simulink model "ex3"  (R2020a)
settings: Solver=ode45  StartTime=0.0  StopTime=8  RelTol=1e-3  EnableMultiTasking=on
values from neighbouring files (symbols this model uses):
  A = gss.a    [ex3.m]
  B = gss.b    [ex3.m]
  C = gss.c    [ex3.m]
  K = place(Aa,Ba,[-4 -5 -7])    [ex3.m]
  L = place(A',C',obsepoles)'    [ex3.m]
settings Model: Creator=Xrisostomos  LastModifiedBy=xriso
settings DataIOCC: LimitDataPoints=on  SaveFormat=Array  ReturnWorkspaceOutputs=off
settings OptimizationCC: LifeSpan=inf
settings DebuggingCC: SFUnexpectedBacktrackingDiag=warning  SFNoUnconditionalDefaultTransitionDiag=warning  SFExecutionAtInitializationDiag=none  ArithmeticOperatorsInVariantConditions=warning
settings HardwareCC: ProdBitPerPointer=32  ProdBitPerSizeT=32  ProdBitPerPtrDiffT=32  ProdLargestAtomicFloat=None  ProdIntDivRoundTo=Undefined  ProdEndianess=Unspecified  ProdWordSize=32  ProdHWDeviceType=32-bit Generic
settings ModelReferenceCC: PropagateSignalLabelsOutOfModel=off
settings SFSimCC: SimUseLocalCustomCode=off  CustomCodeUndefinedFunction=UseInterfaceOnly
settings RTWCC: RTWUseLocalCustomCode=off
settings CodeAppCC: StateflowObjectComments=on
settings GRTTargetCC: TargetLangStandard=C89/C90 (ANSI)
settings ConfigComp: CovMetricSettings=dw  CovHtmlReporting=on  CovSaveCumulativeToWorkspaceVar=on  CovSaveSingleToWorkspaceVar=on  CovExternalEMLEnable=off

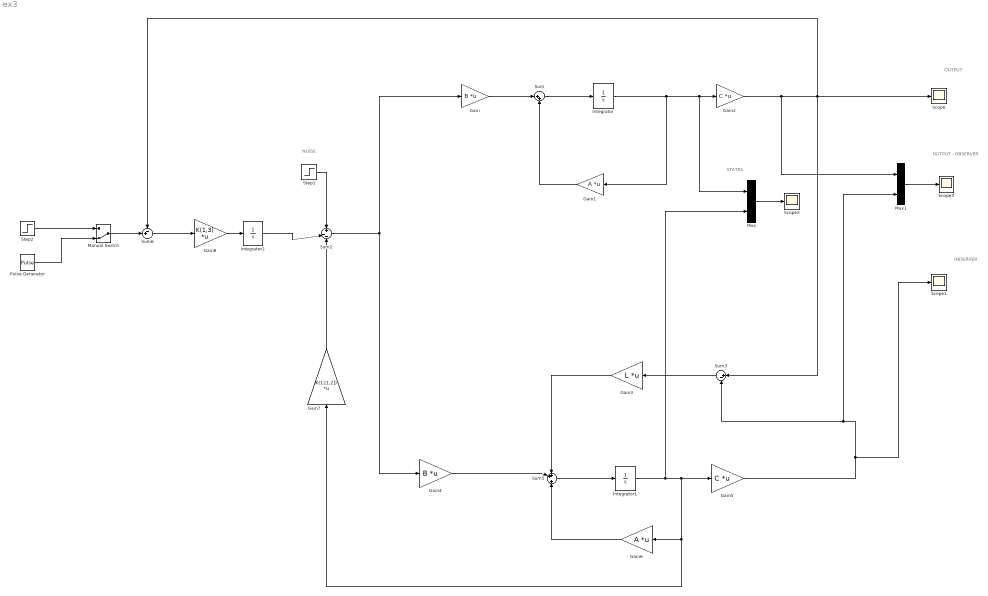
== system ex3 ==
  note: NOISE
  note: OUTPUT
  note: OBSERVER
  note: OUTPUT - OBSERVER
  note: STATES
  Gain : Gain  Gain=B  Multiplication=Matrix(K*u)
  Gain1 : Gain  Gain=A  Multiplication=Matrix(K*u)
  Gain2 : Gain  Gain=C  Multiplication=Matrix(K*u)
  Gain3 : Gain  Gain=L  Multiplication=Matrix(K*u)
  Gain4 : Gain  Gain=B  Multiplication=Matrix(K*u)
  Gain5 : Gain  Gain=C  Multiplication=Matrix(K*u)
  Gain6 : Gain  Gain=A  Multiplication=Matrix(K*u)
  Gain7 : Gain  Gain=K(1,[1,2])  Multiplication=Matrix(K*u)
  Gain8 : Gain  Gain=K(1,3)  Multiplication=Matrix(K*u)
  Integrator : Integrator  InitialCondition=[1 1]
  Integrator1 : Integrator  InitialCondition=[0 0]
  Integrator2 : Integrator
  Manual Switch : ManualSwitch  CurrentSetting=0
  Mux : Mux  Inputs=2
  Mux1 : Mux  Inputs=2
  Pulse Generator : DiscretePulseGenerator  PulseType=Time based  Period=4  PulseWidth=50
  Scope{,1..3} (4 alike) : Scope
  Step1 : Step  Time=5  SampleTime=0
  Step2 : Step  SampleTime=0
  Sum : Sum  Inputs=|++
  Sum2 : Sum  Inputs=+|--
  Sum3 : Sum  Inputs=|+-
  Sum5 : Sum  Inputs=++|+
  Sum6 : Sum  Inputs=-+|
  wires:
  Gain/1 -> Sum/1
  Sum/1 -> Integrator/1
  Integrator/1 -> Mux/1, Gain2/1, Gain1/1
  Gain1/1 -> Sum/2
  Gain3/1 -> Sum5/1
  Sum3/1 -> Gain3/1
  Gain5/1 -> Mux1/2, Sum3/2, Scope1/1
  Gain4/1 -> Sum5/2
  Sum5/1 -> Integrator1/1
  Gain6/1 -> Sum5/3
  Integrator1/1 -> Mux/2, Gain6/1, Gain7/1, Gain5/1
  Sum2/1 -> Gain/1, Gain4/1
  Gain7/1 -> Sum2/3
  Integrator2/1 -> Sum2/2
  Gain8/1 -> Integrator2/1
  Gain2/1 -> Mux1/1, Scope/1, Sum3/1, Sum6/1
  Sum6/1 -> Gain8/1
  Mux/1 -> Scope2/1
  Step1/1 -> Sum2/1
  Mux1/1 -> Scope3/1
  Step2/1 -> Manual Switch/1
  Pulse Generator/1 -> Manual Switch/2
  Manual Switch/1 -> Sum6/2
